simulink model "PID"  (R2020b)
settings: Solver=VariableStepAuto  StartTime=0.0  StopTime=Ts  RelTol=1e-3
values from neighbouring files (symbols this model uses):
  b = 1    [params.m]
  c = 1    [params.m]
  Kc = 3    [params.m]
  Kd = 0.1    [params.m]
  Kff = 1    [params.m]
  Ki = 1    [params.m]
  Kp = 1    [params.m]
  Kpd = 1    [params.m]
  Kpi = 0.2    [params.m]
  Tf = 1    [params.m]
  Tfa1 = 1    [params.m]
  Tfa2 = 1    [params.m]
  Tff1 = 1    [params.m]
  Tff2 = 3    [params.m]
  Ts = 100    [params.m]
  u_max = 5    [params.m]
  u_min = -5    [params.m]
  y_zad = 5    [params.m]
  z_zad = 2    [params.m]
libraries: pid_lib x6
settings Model: Creator=micha  LastModifiedBy=micha
settings DebuggingCC: IgnoredZcDiagnostic=error

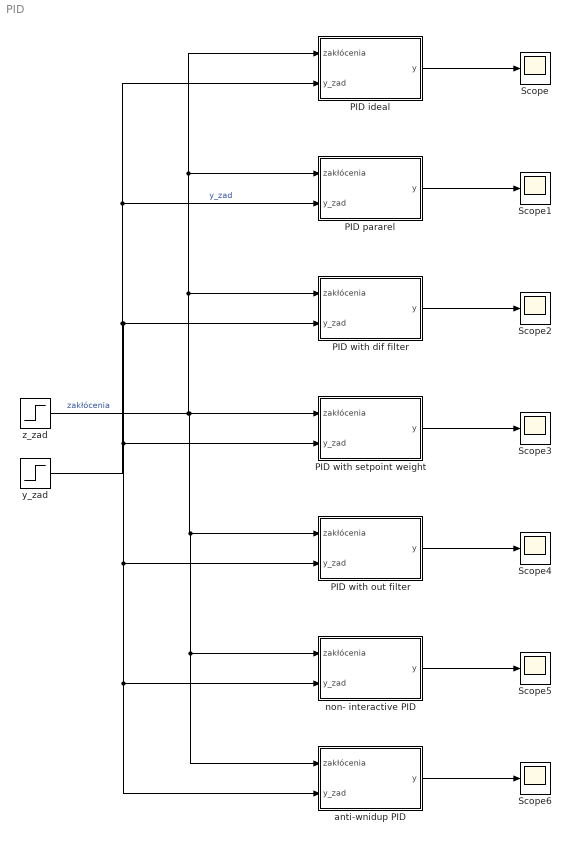
== system PID ==
  PID ideal : Subsystem
  PID pararel : Subsystem
  PID with dif filter : Subsystem
  "PID with out filter " : Subsystem
  PID with setpoint weight : Subsystem
  Scope{,1..6} (7 alike) : Scope
  anti-wnidup PID : Subsystem
  non- interactive PID : Subsystem
  y_zad : Step  After=y_zad  SampleTime=1
  z_zad : Step  Time=50  After=z_zad  SampleTime=1
  wires:
  PID ideal/1(y) -> Scope/1
  PID pararel/1(y) -> Scope1/1
  PID with dif filter/1(y) -> Scope2/1
  PID with setpoint weight/1(y) -> Scope3/1
  "PID with out filter "/1(y) -> Scope4/1
  z_zad/1 -> PID ideal/1(zakłócenia), PID pararel/1(zakłócenia), PID with dif filter/1(zakłócenia), anti-wnidup PID/1(zakłócenia), non- interactive PID/1(zakłócenia), "PID with out filter "/1(zakłócenia), PID with setpoint weight/1(zakłócenia)  "zakłócenia"
  y_zad/1 -> PID ideal/2(y_zad), PID pararel/2(y_zad), anti-wnidup PID/2(y_zad), non- interactive PID/2(y_zad), "PID with out filter "/2(y_zad), PID with setpoint weight/2(y_zad), PID with dif filter/2(y_zad)  "y_zad"
  non- interactive PID/1(y) -> Scope5/1
  anti-wnidup PID/1(y) -> Scope6/1

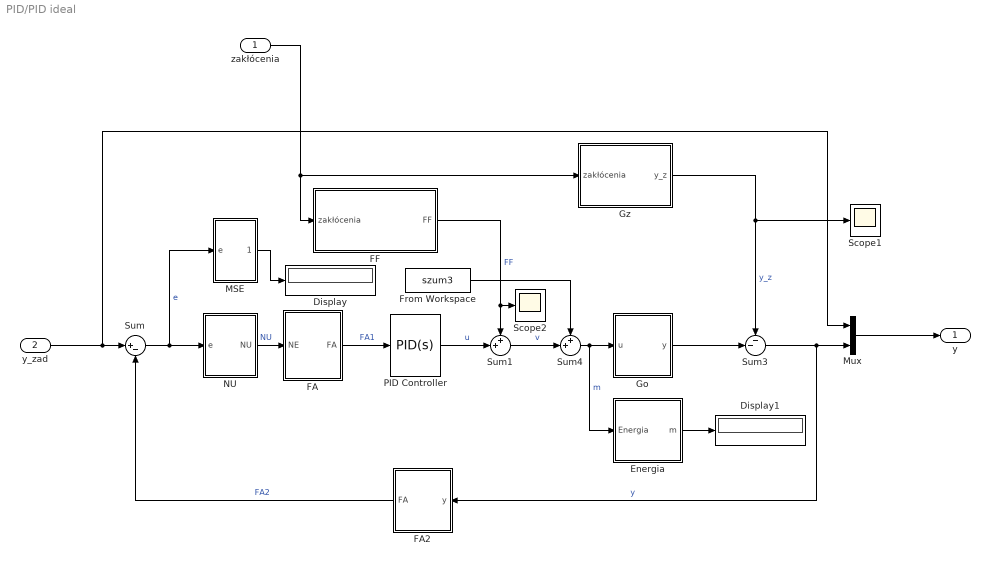
== system PID/PID ideal ==
  zakłócenia : Inport
  y_zad : Inport  Port=2
  Display : Display
  Display1 : Display
  Energia : Subsystem
  FA : Subsystem
  FA2 : Subsystem
  FF : Subsystem
  From Workspace : FromWorkspace  VariableName=szum3  OutDataTypeStr=double  SampleTime=1
  Go : Subsystem
  Gz : Subsystem
  MSE : Subsystem
  Mux : Mux  Inputs=2
  NU : Subsystem
  PID Controller : pid_lib/PID Controller  Controller=PID  Form=Ideal  TimeDomain=Continuous-time  UseExternalTs=off  SampleTime=-1  IntegratorMethod=Forward Euler  FilterMethod=Forward Euler  ControllerParametersSource=internal  P=1.05779168543042  I=0.244759575952049  D=0.993541953243631  UseFilter=on  N=1  TunerSelectOption=Transfer Function Based (PID Tuner App)  InitialConditionSource=internal  InitialConditionForIntegrator=0  InitialConditionForFilter=0  DifferentiatorICPrevScaledInput=0  ExternalReset=none  TrackingMode=off  Kt=1  LimitOutput=off  SatLimitsSource=internal  UpperSaturationLimit=inf  LowerSaturationLimit=-inf  LinearizeAsGain=on  AntiWindupMode=none  Kb=1  POutMin=[]  POutMax=[]  IOutMin=[]  IOutMax=[]  DOutMin=[]  DOutMax=[]  NOutMin=[]  NOutMax=[]  SumOutMin=[]  SumOutMax=[]  SaturationOutMin=[]  SaturationOutMax=[]  PParamMin=[]  PParamMax=[]  IParamMin=[]  IParamMax=[]  DParamMin=[]  DParamMax=[]  NParamMin=[]  NParamMax=[]  KbParamMin=[]  KbParamMax=[]  KtParamMin=[]  KtParamMax=[]  KbOutMin=[]  KbOutMax=[]  KtOutMin=[]  KtOutMax=[]  IntegratorOutMin=[]  IntegratorOutMax=[]  FilterOutMin=[]  FilterOutMax=[]  SumI1OutMin=[]  SumI1OutMax=[]  SumI2OutMin=[]  SumI2OutMax=[]  SumI3OutMin=[]  SumI3OutMax=[]  SumI4OutMin=[]  SumI4OutMax=[]  SumDOutMin=[]  SumDOutMax=[]  DifferentiatorOutMin=[]  DifferentiatorOutMax=[]  FilterDiffOutCoefMin=[]  FilterDiffOutCoefMax=[]  ReciprocalOutMin=[]  ReciprocalOutMax=[]  SumDenOutMin=[]  SumDenOutMax=[]  SumNumOutMin=[]  SumNumOutMax=[]  DivideOutMin=[]  DivideOutMax=[]  UdiffTsProdOutMin=[]  UdiffTsProdOutMax=[]  NTsProdOutMin=[]  NTsProdOutMax=[]  UintegralTsProdOutMin=[]  UintegralTsProdOutMax=[]  UngainTsProdOutMin=[]  UngainTsProdOutMax=[]  IntegratorContinuousStateAttributes=''  IntegratorStateMustResolveToSignalObject=off  IntegratorRTWStateStorageClass=Auto  FilterContinuousStateAttributes=''  FilterStateMustResolveToSignalObject=off  FilterRTWStateStorageClass=Auto  ParallelPVariant=Passthrough  IdealPVariant=InternalParameters  IVariant=InternalParameters  DVariant=InternalParameters  IntegratorVariant=Continuous  SatVariant=Disabled  AWVariant=Passthrough  PCopyVariant=Disabled  TRVariant=Disabled  FdbkBlocksVariant=Forward  IdealPFdbkVariant=Disabled  SatFdbkVariant=Disabled  DerivativeFilterVariant=ContFilter  NVariant=InternalParameters  NCopyVariant=Disabled  FilterICVariant=InternalICsFilter  IntegratorICVariant=InternalICs  ExternalResetVariant=Disabled  TRSumVariant=Passthrough  SumFdbkVariant=Disabled  SumVariant=Sum_PID  TsampFilterVariant=InternalTs  TsampNgainVariant=Passthrough  TsampIntegralVariant=Passthrough  ExternalSaturationOutDataTypeStr=Inherit: Same as second input
  Scope1 : Scope
  Scope2 : Scope
  Sum : Sum  Inputs=|+-
  Sum1 : Sum  Inputs=++|
  Sum3 : Sum  Inputs=--|
  Sum4 : Sum  Inputs=++|
  y : Outport
  wires:
  Sum/1 -> MSE/1(e), NU/1(e)  "e"
  Sum3/1 -> FA2/1(y), Mux/2  "y"
  Gz/1(y_z) -> Scope1/1, Sum3/1  "y_z"
  Energia/1(m) -> Display1/1
  Sum4/1 -> Energia/1(Energia), Go/1(u)  "m"
  zakłócenia/1 -> FF/1(zakłócenia), Gz/1(zakłócenia)
  MSE/1(MSE) -> Display/1
  Go/1(y) -> Sum3/2
  PID Controller/1 -> Sum1/2  "u"
  Sum1/1 -> Sum4/2  "v"
  Mux/1 -> y/1
  y_zad/1 -> Mux/1, Sum/1
  FF/1(FF) -> Scope2/1, Sum1/1  "FF"
  FA/1(FA) -> PID Controller/1  "FA1"
  FA2/1(FA) -> Sum/2  "FA2"
  NU/1(NU) -> FA/1(NE)  "NU"
  From Workspace/1 -> Sum4/1

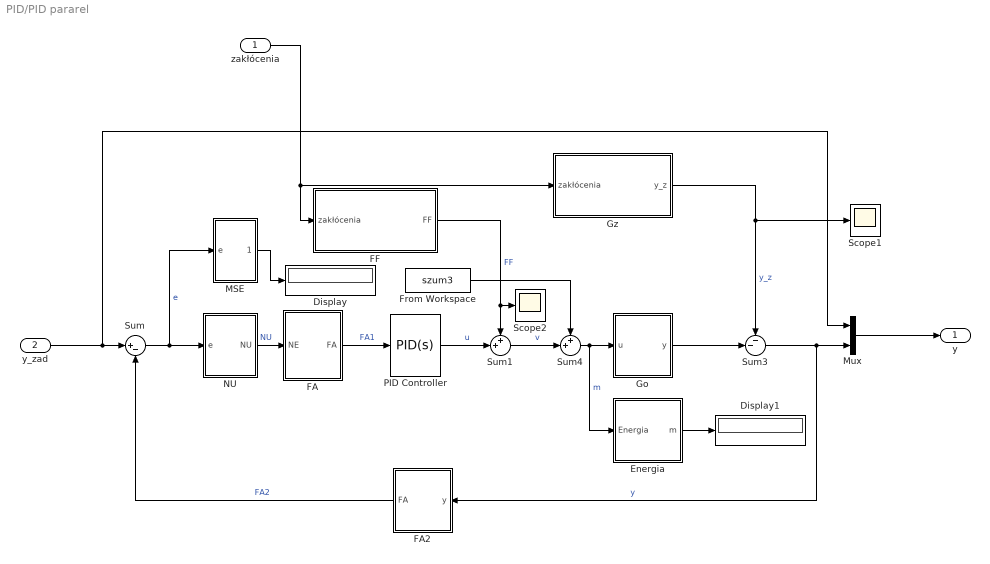
== system PID/PID pararel ==
  zakłócenia : Inport
  y_zad : Inport  Port=2
  Display : Display
  Display1 : Display
  Energia : Subsystem
  FA : Subsystem
  FA2 : Subsystem
  FF : Subsystem
  From Workspace : FromWorkspace  VariableName=szum3  OutDataTypeStr=double  SampleTime=1
  Go : Subsystem
  Gz : Subsystem
  MSE : Subsystem
  Mux : Mux  Inputs=2
  NU : Subsystem
  PID Controller : pid_lib/PID Controller  Controller=PID  Form=Parallel  TimeDomain=Continuous-time  UseExternalTs=off  SampleTime=-1  IntegratorMethod=Forward Euler  FilterMethod=Forward Euler  ControllerParametersSource=internal  P=1.05779168543042  I=0.258904644371552  D=1.05096041726741  UseFilter=on  N=1  TunerSelectOption=Transfer Function Based (PID Tuner App)  InitialConditionSource=internal  InitialConditionForIntegrator=0  InitialConditionForFilter=0  DifferentiatorICPrevScaledInput=0  ExternalReset=none  TrackingMode=off  Kt=1  LimitOutput=off  SatLimitsSource=internal  UpperSaturationLimit=inf  LowerSaturationLimit=-inf  LinearizeAsGain=on  AntiWindupMode=none  Kb=1  POutMin=[]  POutMax=[]  IOutMin=[]  IOutMax=[]  DOutMin=[]  DOutMax=[]  NOutMin=[]  NOutMax=[]  SumOutMin=[]  SumOutMax=[]  SaturationOutMin=[]  SaturationOutMax=[]  PParamMin=[]  PParamMax=[]  IParamMin=[]  IParamMax=[]  DParamMin=[]  DParamMax=[]  NParamMin=[]  NParamMax=[]  KbParamMin=[]  KbParamMax=[]  KtParamMin=[]  KtParamMax=[]  KbOutMin=[]  KbOutMax=[]  KtOutMin=[]  KtOutMax=[]  IntegratorOutMin=[]  IntegratorOutMax=[]  FilterOutMin=[]  FilterOutMax=[]  SumI1OutMin=[]  SumI1OutMax=[]  SumI2OutMin=[]  SumI2OutMax=[]  SumI3OutMin=[]  SumI3OutMax=[]  SumI4OutMin=[]  SumI4OutMax=[]  SumDOutMin=[]  SumDOutMax=[]  DifferentiatorOutMin=[]  DifferentiatorOutMax=[]  FilterDiffOutCoefMin=[]  FilterDiffOutCoefMax=[]  ReciprocalOutMin=[]  ReciprocalOutMax=[]  SumDenOutMin=[]  SumDenOutMax=[]  SumNumOutMin=[]  SumNumOutMax=[]  DivideOutMin=[]  DivideOutMax=[]  UdiffTsProdOutMin=[]  UdiffTsProdOutMax=[]  NTsProdOutMin=[]  NTsProdOutMax=[]  UintegralTsProdOutMin=[]  UintegralTsProdOutMax=[]  UngainTsProdOutMin=[]  UngainTsProdOutMax=[]  IntegratorContinuousStateAttributes=''  IntegratorStateMustResolveToSignalObject=off  IntegratorRTWStateStorageClass=Auto  FilterContinuousStateAttributes=''  FilterStateMustResolveToSignalObject=off  FilterRTWStateStorageClass=Auto  ParallelPVariant=InternalParameters  IdealPVariant=Disabled  IVariant=InternalParameters  DVariant=InternalParameters  IntegratorVariant=Continuous  SatVariant=Disabled  AWVariant=Passthrough  PCopyVariant=Disabled  TRVariant=Disabled  FdbkBlocksVariant=Forward  IdealPFdbkVariant=Disabled  SatFdbkVariant=Disabled  DerivativeFilterVariant=ContFilter  NVariant=InternalParameters  NCopyVariant=Disabled  FilterICVariant=InternalICsFilter  IntegratorICVariant=InternalICs  ExternalResetVariant=Disabled  TRSumVariant=Passthrough  SumFdbkVariant=Disabled  SumVariant=Sum_PID  TsampFilterVariant=InternalTs  TsampNgainVariant=Passthrough  TsampIntegralVariant=Passthrough  ExternalSaturationOutDataTypeStr=Inherit: Same as second input
  Scope1 : Scope
  Scope2 : Scope
  Sum : Sum  Inputs=|+-
  Sum1 : Sum  Inputs=++|
  Sum3 : Sum  Inputs=--|
  Sum4 : Sum  Inputs=++|
  y : Outport
  wires:
  Sum/1 -> MSE/1(e), NU/1(e)  "e"
  Sum3/1 -> FA2/1(y), Mux/2  "y"
  Gz/1(y_z) -> Scope1/1, Sum3/1  "y_z"
  Energia/1(m) -> Display1/1
  From Workspace/1 -> Sum4/1
  Sum4/1 -> Energia/1(Energia), Go/1(u)  "m"
  zakłócenia/1 -> FF/1(zakłócenia), Gz/1(zakłócenia)
  MSE/1(MSE) -> Display/1
  Go/1(y) -> Sum3/2
  PID Controller/1 -> Sum1/2  "u"
  Sum1/1 -> Sum4/2  "v"
  Mux/1 -> y/1
  y_zad/1 -> Mux/1, Sum/1
  FF/1(FF) -> Scope2/1, Sum1/1  "FF"
  FA/1(FA) -> PID Controller/1  "FA1"
  FA2/1(FA) -> Sum/2  "FA2"
  NU/1(NU) -> FA/1(NE)  "NU"

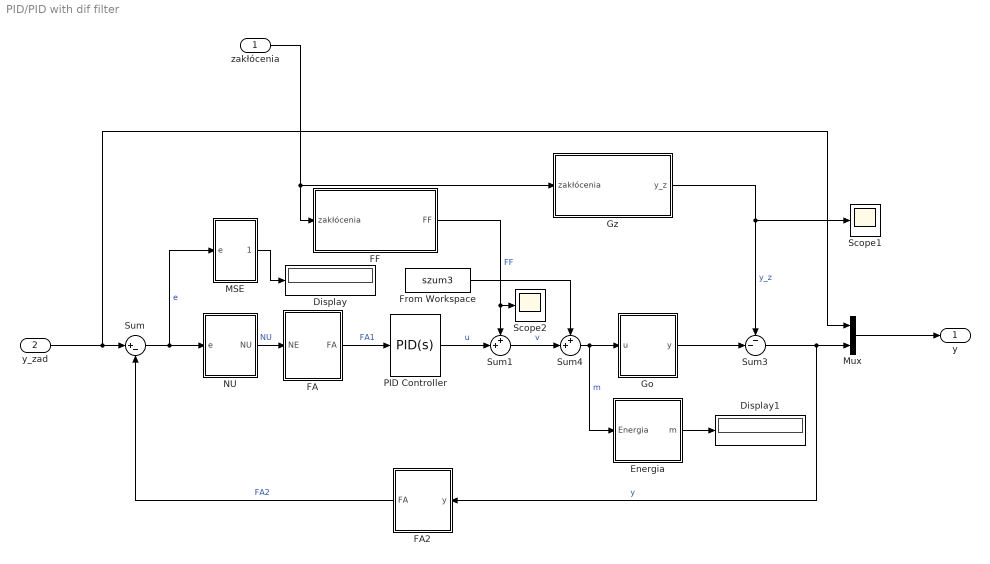
== system PID/PID with dif filter ==
  zakłócenia : Inport
  y_zad : Inport  Port=2
  Display : Display
  Display1 : Display
  Energia : Subsystem
  FA : Subsystem
  FA2 : Subsystem
  FF : Subsystem
  From Workspace : FromWorkspace  VariableName=szum3  OutDataTypeStr=double  SampleTime=1
  Go : Subsystem
  Gz : Subsystem
  MSE : Subsystem
  Mux : Mux  Inputs=2
  NU : Subsystem
  PID Controller : pid_lib/PID Controller  Controller=PID  Form=Ideal  TimeDomain=Continuous-time  UseExternalTs=off  SampleTime=-1  IntegratorMethod=Forward Euler  FilterMethod=Forward Euler  ControllerParametersSource=internal  P=1.05779168543042  I=0.244759575952049  D=0.993541953243631  UseFilter=on  N=49.2140953621087  TunerSelectOption=Transfer Function Based (PID Tuner App)  InitialConditionSource=internal  InitialConditionForIntegrator=0  InitialConditionForFilter=0  DifferentiatorICPrevScaledInput=0  ExternalReset=none  TrackingMode=off  Kt=1  LimitOutput=off  SatLimitsSource=internal  UpperSaturationLimit=inf  LowerSaturationLimit=-inf  LinearizeAsGain=on  AntiWindupMode=none  Kb=1  POutMin=[]  POutMax=[]  IOutMin=[]  IOutMax=[]  DOutMin=[]  DOutMax=[]  NOutMin=[]  NOutMax=[]  SumOutMin=[]  SumOutMax=[]  SaturationOutMin=[]  SaturationOutMax=[]  PParamMin=[]  PParamMax=[]  IParamMin=[]  IParamMax=[]  DParamMin=[]  DParamMax=[]  NParamMin=[]  NParamMax=[]  KbParamMin=[]  KbParamMax=[]  KtParamMin=[]  KtParamMax=[]  KbOutMin=[]  KbOutMax=[]  KtOutMin=[]  KtOutMax=[]  IntegratorOutMin=[]  IntegratorOutMax=[]  FilterOutMin=[]  FilterOutMax=[]  SumI1OutMin=[]  SumI1OutMax=[]  SumI2OutMin=[]  SumI2OutMax=[]  SumI3OutMin=[]  SumI3OutMax=[]  SumI4OutMin=[]  SumI4OutMax=[]  SumDOutMin=[]  SumDOutMax=[]  DifferentiatorOutMin=[]  DifferentiatorOutMax=[]  FilterDiffOutCoefMin=[]  FilterDiffOutCoefMax=[]  ReciprocalOutMin=[]  ReciprocalOutMax=[]  SumDenOutMin=[]  SumDenOutMax=[]  SumNumOutMin=[]  SumNumOutMax=[]  DivideOutMin=[]  DivideOutMax=[]  UdiffTsProdOutMin=[]  UdiffTsProdOutMax=[]  NTsProdOutMin=[]  NTsProdOutMax=[]  UintegralTsProdOutMin=[]  UintegralTsProdOutMax=[]  UngainTsProdOutMin=[]  UngainTsProdOutMax=[]  IntegratorContinuousStateAttributes=''  IntegratorStateMustResolveToSignalObject=off  IntegratorRTWStateStorageClass=Auto  FilterContinuousStateAttributes=''  FilterStateMustResolveToSignalObject=off  FilterRTWStateStorageClass=Auto  ParallelPVariant=Passthrough  IdealPVariant=InternalParameters  IVariant=InternalParameters  DVariant=InternalParameters  IntegratorVariant=Continuous  SatVariant=Disabled  AWVariant=Passthrough  PCopyVariant=Disabled  TRVariant=Disabled  FdbkBlocksVariant=Forward  IdealPFdbkVariant=Disabled  SatFdbkVariant=Disabled  DerivativeFilterVariant=ContFilter  NVariant=InternalParameters  NCopyVariant=Disabled  FilterICVariant=InternalICsFilter  IntegratorICVariant=InternalICs  ExternalResetVariant=Disabled  TRSumVariant=Passthrough  SumFdbkVariant=Disabled  SumVariant=Sum_PID  TsampFilterVariant=InternalTs  TsampNgainVariant=Passthrough  TsampIntegralVariant=Passthrough  ExternalSaturationOutDataTypeStr=Inherit: Same as second input
  Scope1 : Scope
  Scope2 : Scope
  Sum : Sum  Inputs=|+-
  Sum1 : Sum  Inputs=++|
  Sum3 : Sum  Inputs=--|
  Sum4 : Sum  Inputs=++|
  y : Outport
  wires:
  Sum/1 -> MSE/1(e), NU/1(e)  "e"
  Sum3/1 -> FA2/1(y), Mux/2  "y"
  Gz/1(y_z) -> Scope1/1, Sum3/1  "y_z"
  Energia/1(m) -> Display1/1
  From Workspace/1 -> Sum4/1
  Sum4/1 -> Energia/1(Energia), Go/1(u)  "m"
  zakłócenia/1 -> FF/1(zakłócenia), Gz/1(zakłócenia)
  MSE/1(MSE) -> Display/1
  Go/1(y) -> Sum3/2
  PID Controller/1 -> Sum1/2  "u"
  Sum1/1 -> Sum4/2  "v"
  Mux/1 -> y/1
  y_zad/1 -> Mux/1, Sum/1
  FF/1(FF) -> Scope2/1, Sum1/1  "FF"
  FA/1(FA) -> PID Controller/1  "FA1"
  FA2/1(FA) -> Sum/2  "FA2"
  NU/1(NU) -> FA/1(NE)  "NU"

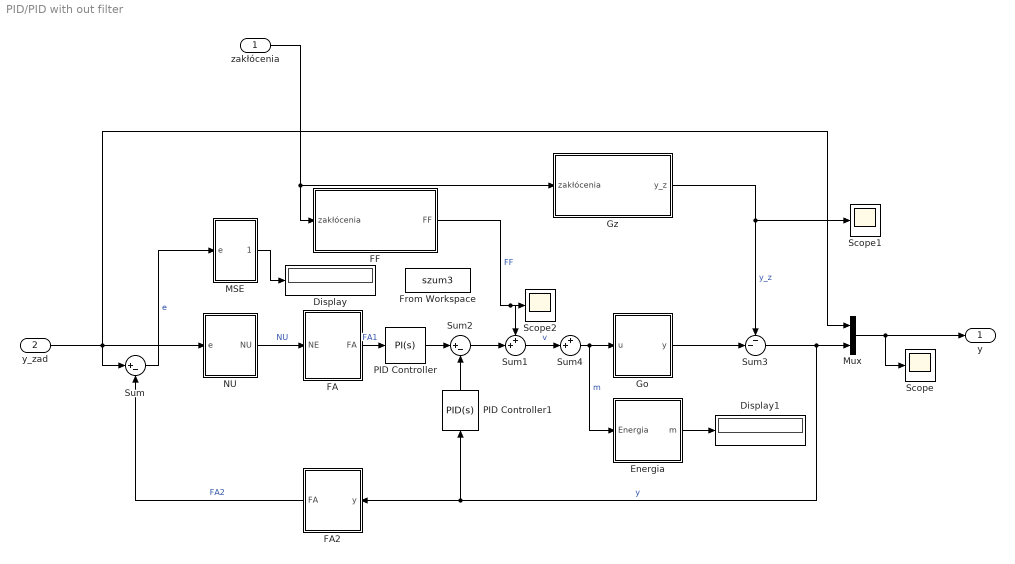
== system PID/PID with out filter  ==
  zakłócenia : Inport
  y_zad : Inport  Port=2
  Display : Display
  Display1 : Display
  Energia : Subsystem
  FA : Subsystem
  FA2 : Subsystem
  FF : Subsystem
  From Workspace : FromWorkspace  VariableName=szum3  OutDataTypeStr=double  SampleTime=1
  Go : Subsystem
  Gz : Subsystem
  MSE : Subsystem
  Mux : Mux  Inputs=2
  NU : Subsystem
  PID Controller : pid_lib/PID Controller  Controller=PI  Form=Parallel  TimeDomain=Continuous-time  UseExternalTs=off  SampleTime=-1  IntegratorMethod=Forward Euler  FilterMethod=Forward Euler  ControllerParametersSource=internal  P=1.5  I=0.38  D=0  UseFilter=on  N=100  TunerSelectOption=Transfer Function Based (PID Tuner App)  InitialConditionSource=internal  InitialConditionForIntegrator=0  InitialConditionForFilter=0  DifferentiatorICPrevScaledInput=0  ExternalReset=none  TrackingMode=off  Kt=1  LimitOutput=off  SatLimitsSource=internal  UpperSaturationLimit=inf  LowerSaturationLimit=-inf  LinearizeAsGain=on  AntiWindupMode=none  Kb=1  POutMin=[]  POutMax=[]  IOutMin=[]  IOutMax=[]  DOutMin=[]  DOutMax=[]  NOutMin=[]  NOutMax=[]  SumOutMin=[]  SumOutMax=[]  SaturationOutMin=[]  SaturationOutMax=[]  PParamMin=[]  PParamMax=[]  IParamMin=[]  IParamMax=[]  DParamMin=[]  DParamMax=[]  NParamMin=[]  NParamMax=[]  KbParamMin=[]  KbParamMax=[]  KtParamMin=[]  KtParamMax=[]  KbOutMin=[]  KbOutMax=[]  KtOutMin=[]  KtOutMax=[]  IntegratorOutMin=[]  IntegratorOutMax=[]  FilterOutMin=[]  FilterOutMax=[]  SumI1OutMin=[]  SumI1OutMax=[]  SumI2OutMin=[]  SumI2OutMax=[]  SumI3OutMin=[]  SumI3OutMax=[]  SumI4OutMin=[]  SumI4OutMax=[]  SumDOutMin=[]  SumDOutMax=[]  DifferentiatorOutMin=[]  DifferentiatorOutMax=[]  FilterDiffOutCoefMin=[]  FilterDiffOutCoefMax=[]  ReciprocalOutMin=[]  ReciprocalOutMax=[]  SumDenOutMin=[]  SumDenOutMax=[]  SumNumOutMin=[]  SumNumOutMax=[]  DivideOutMin=[]  DivideOutMax=[]  UdiffTsProdOutMin=[]  UdiffTsProdOutMax=[]  NTsProdOutMin=[]  NTsProdOutMax=[]  UintegralTsProdOutMin=[]  UintegralTsProdOutMax=[]  UngainTsProdOutMin=[]  UngainTsProdOutMax=[]  IntegratorContinuousStateAttributes=''  IntegratorStateMustResolveToSignalObject=off  IntegratorRTWStateStorageClass=Auto  FilterContinuousStateAttributes=''  FilterStateMustResolveToSignalObject=off  FilterRTWStateStorageClass=Auto  ParallelPVariant=InternalParameters  IdealPVariant=Disabled  IVariant=InternalParameters  DVariant=Disabled  IntegratorVariant=Continuous  SatVariant=Disabled  AWVariant=Passthrough  PCopyVariant=Disabled  TRVariant=Disabled  FdbkBlocksVariant=Forward  IdealPFdbkVariant=Disabled  SatFdbkVariant=Disabled  DerivativeFilterVariant=Disabled  NVariant=Disabled  NCopyVariant=Disabled_SignalSpec  FilterICVariant=Disabled  IntegratorICVariant=InternalICs  ExternalResetVariant=Disabled  TRSumVariant=Passthrough  SumFdbkVariant=Disabled  SumVariant=Sum_PI  TsampFilterVariant=InternalTs  TsampNgainVariant=Passthrough  TsampIntegralVariant=Passthrough  ExternalSaturationOutDataTypeStr=Inherit: Same as second input
  PID Controller1 : pid_lib/PID Controller  Controller=PID  Form=Parallel  TimeDomain=Continuous-time  UseExternalTs=off  SampleTime=-1  IntegratorMethod=Forward Euler  FilterMethod=Forward Euler  ControllerParametersSource=internal  P=0.668790156897551  I=0.381936066634179  D=-0.0850078103169395  UseFilter=on  N=1.08026904337961  TunerSelectOption=Transfer Function Based (PID Tuner App)  InitialConditionSource=internal  InitialConditionForIntegrator=0  InitialConditionForFilter=0  DifferentiatorICPrevScaledInput=0  ExternalReset=none  TrackingMode=off  Kt=1  LimitOutput=off  SatLimitsSource=internal  UpperSaturationLimit=inf  LowerSaturationLimit=-inf  LinearizeAsGain=on  AntiWindupMode=none  Kb=1  POutMin=[]  POutMax=[]  IOutMin=[]  IOutMax=[]  DOutMin=[]  DOutMax=[]  NOutMin=[]  NOutMax=[]  SumOutMin=[]  SumOutMax=[]  SaturationOutMin=[]  SaturationOutMax=[]  PParamMin=[]  PParamMax=[]  IParamMin=[]  IParamMax=[]  DParamMin=[]  DParamMax=[]  NParamMin=[]  NParamMax=[]  KbParamMin=[]  KbParamMax=[]  KtParamMin=[]  KtParamMax=[]  KbOutMin=[]  KbOutMax=[]  KtOutMin=[]  KtOutMax=[]  IntegratorOutMin=[]  IntegratorOutMax=[]  FilterOutMin=[]  FilterOutMax=[]  SumI1OutMin=[]  SumI1OutMax=[]  SumI2OutMin=[]  SumI2OutMax=[]  SumI3OutMin=[]  SumI3OutMax=[]  SumI4OutMin=[]  SumI4OutMax=[]  SumDOutMin=[]  SumDOutMax=[]  DifferentiatorOutMin=[]  DifferentiatorOutMax=[]  FilterDiffOutCoefMin=[]  FilterDiffOutCoefMax=[]  ReciprocalOutMin=[]  ReciprocalOutMax=[]  SumDenOutMin=[]  SumDenOutMax=[]  SumNumOutMin=[]  SumNumOutMax=[]  DivideOutMin=[]  DivideOutMax=[]  UdiffTsProdOutMin=[]  UdiffTsProdOutMax=[]  NTsProdOutMin=[]  NTsProdOutMax=[]  UintegralTsProdOutMin=[]  UintegralTsProdOutMax=[]  UngainTsProdOutMin=[]  UngainTsProdOutMax=[]  IntegratorContinuousStateAttributes=''  IntegratorStateMustResolveToSignalObject=off  IntegratorRTWStateStorageClass=Auto  FilterContinuousStateAttributes=''  FilterStateMustResolveToSignalObject=off  FilterRTWStateStorageClass=Auto  ParallelPVariant=InternalParameters  IdealPVariant=Disabled  IVariant=InternalParameters  DVariant=InternalParameters  IntegratorVariant=Continuous  SatVariant=Disabled  AWVariant=Passthrough  PCopyVariant=Disabled  TRVariant=Disabled  FdbkBlocksVariant=Forward  IdealPFdbkVariant=Disabled  SatFdbkVariant=Disabled  DerivativeFilterVariant=ContFilter  NVariant=InternalParameters  NCopyVariant=Disabled  FilterICVariant=InternalICsFilter  IntegratorICVariant=InternalICs  ExternalResetVariant=Disabled  TRSumVariant=Passthrough  SumFdbkVariant=Disabled  SumVariant=Sum_PID  TsampFilterVariant=InternalTs  TsampNgainVariant=Passthrough  TsampIntegralVariant=Passthrough  ExternalSaturationOutDataTypeStr=Inherit: Same as second input
  Scope : Scope
  Scope1 : Scope
  Scope2 : Scope
  Sum : Sum  Inputs=|+-
  Sum1 : Sum  Inputs=++|
  Sum2 : Sum  Inputs=|+-
  Sum3 : Sum  Inputs=--|
  Sum4 : Sum  Inputs=++|
  y : Outport
  wires:
  Sum/1 -> MSE/1(e)  "e"
  Sum3/1 -> PID Controller1/1, FA2/1(y), Mux/2  "y"
  Gz/1(y_z) -> Scope1/1, Sum3/1  "y_z"
  Energia/1(m) -> Display1/1
  Sum4/1 -> Go/1(u), Energia/1(Energia)  "m"
  zakłócenia/1 -> FF/1(zakłócenia), Gz/1(zakłócenia)
  MSE/1(MSE) -> Display/1
  Go/1(y) -> Sum3/2
  Sum1/1 -> Sum4/2  "v"
  Mux/1 -> Scope/1, y/1
  y_zad/1 -> Mux/1, Sum/1, NU/1(e)
  FF/1(FF) -> Scope2/1, Sum1/1  "FF"
  FA/1(FA) -> PID Controller/1  "FA1"
  FA2/1(FA) -> Sum/2  "FA2"
  NU/1(NU) -> FA/1(NE)  "NU"
  Sum2/1 -> Sum1/2
  PID Controller/1 -> Sum2/1
  PID Controller1/1 -> Sum2/2

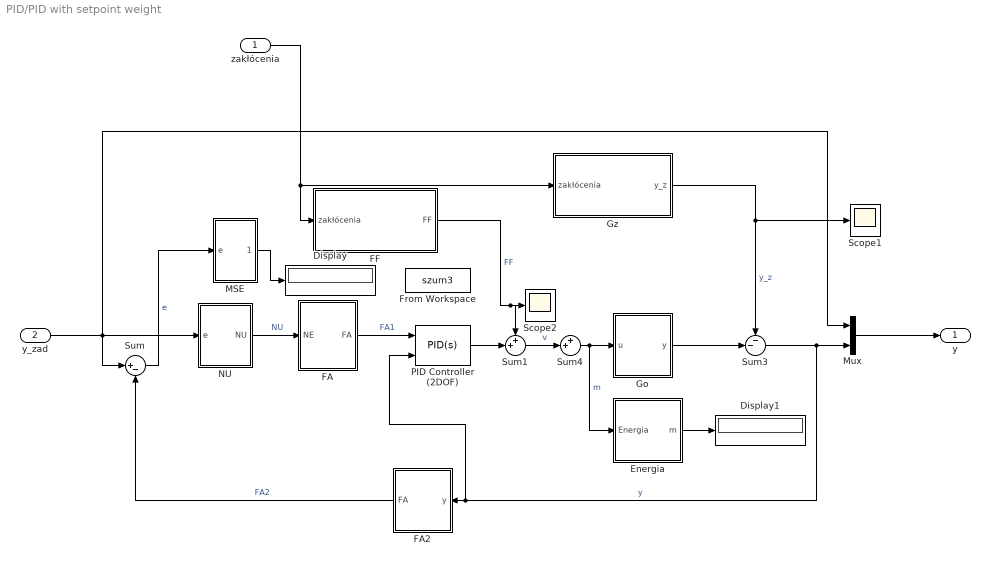
== system PID/PID with setpoint weight ==
  zakłócenia : Inport
  y_zad : Inport  Port=2
  Display : Display
  Display1 : Display
  Energia : Subsystem
  FA : Subsystem
  FA2 : Subsystem
  FF : Subsystem
  From Workspace : FromWorkspace  VariableName=szum3  OutDataTypeStr=double  SampleTime=1
  Go : Subsystem
  Gz : Subsystem
  MSE : Subsystem
  Mux : Mux  Inputs=2
  NU : Subsystem
  PID Controller (2DOF) : pid_lib/PID Controller (2DOF)  Controller=PID  Form=Ideal  TimeDomain=Continuous-time  UseExternalTs=off  SampleTime=-1  IntegratorMethod=Forward Euler  FilterMethod=Forward Euler  ControllerParametersSource=internal  P=0.652114055675395  I=0.613314096005047  D=0  UseFilter=on  N=100  b=1  c=1  TunerSelectOption=Transfer Function Based (PID Tuner App)  InitialConditionSource=internal  InitialConditionForIntegrator=0  InitialConditionForFilter=0  DifferentiatorICPrevScaledInput=0  ExternalReset=none  TrackingMode=off  Kt=1  LimitOutput=off  SatLimitsSource=internal  UpperSaturationLimit=inf  LowerSaturationLimit=-inf  LinearizeAsGain=on  AntiWindupMode=none  Kb=1  POutMin=[]  POutMax=[]  IOutMin=[]  IOutMax=[]  DOutMin=[]  DOutMax=[]  NOutMin=[]  NOutMax=[]  bOutMin=[]  bOutMax=[]  cOutMin=[]  cOutMax=[]  SumOutMin=[]  SumOutMax=[]  SaturationOutMin=[]  SaturationOutMax=[]  PParamMin=[]  PParamMax=[]  IParamMin=[]  IParamMax=[]  DParamMin=[]  DParamMax=[]  NParamMin=[]  NParamMax=[]  bParamMin=[]  bParamMax=[]  cParamMin=[]  cParamMax=[]  KbParamMin=[]  KbParamMax=[]  KtParamMin=[]  KtParamMax=[]  KbOutMin=[]  KbOutMax=[]  KtOutMin=[]  KtOutMax=[]  IntegratorOutMin=[]  IntegratorOutMax=[]  FilterOutMin=[]  FilterOutMax=[]  SumI1OutMin=[]  SumI1OutMax=[]  SumI2OutMin=[]  SumI2OutMax=[]  SumI3OutMin=[]  SumI3OutMax=[]  SumI4OutMin=[]  SumI4OutMax=[]  SumDOutMin=[]  SumDOutMax=[]  Sum1OutMin=[]  Sum1OutMax=[]  Sum2OutMin=[]  Sum2OutMax=[]  Sum3OutMin=[]  Sum3OutMax=[]  DifferentiatorOutMin=[]  DifferentiatorOutMax=[]  FilterDiffOutCoefMin=[]  FilterDiffOutCoefMax=[]  ReciprocalOutMin=[]  ReciprocalOutMax=[]  SumDenOutMin=[]  SumDenOutMax=[]  SumNumOutMin=[]  SumNumOutMax=[]  DivideOutMin=[]  DivideOutMax=[]  UdiffTsProdOutMin=[]  UdiffTsProdOutMax=[]  NTsProdOutMin=[]  NTsProdOutMax=[]  UintegralTsProdOutMin=[]  UintegralTsProdOutMax=[]  UngainTsProdOutMin=[]  UngainTsProdOutMax=[]  IntegratorContinuousStateAttributes=''  IntegratorStateMustResolveToSignalObject=off  IntegratorRTWStateStorageClass=Auto  FilterContinuousStateAttributes=''  FilterStateMustResolveToSignalObject=off  FilterRTWStateStorageClass=Auto  ParallelPVariant=Passthrough  IdealPVariant=InternalParameters  IVariant=InternalParameters  DVariant=InternalParameters  bVariant=InternalParameters  cVariant=InternalParameters  IntegratorVariant=Continuous  SatVariant=Disabled  AWVariant=Passthrough  PCopyVariant=Disabled  TRVariant=Disabled  FdbkBlocksVariant=Forward  IdealPFdbkVariant=Disabled  SatFdbkVariant=Disabled  DerivativeFilterVariant=ContFilter  NVariant=InternalParameters  NCopyVariant=Disabled  FilterICVariant=InternalICsFilter  IntegratorICVariant=InternalICs  ExternalResetVariant=Disabled  TRSumVariant=Passthrough  SumFdbkVariant=Disabled  SumVariant=Sum_PID  TsampFilterVariant=InternalTs  TsampNgainVariant=Passthrough  TsampIntegralVariant=Passthrough  ExternalSaturationOutDataTypeStr=Inherit: Same as second input
      settings: SourceProductBaseCode=SL
  Scope1 : Scope
  Scope2 : Scope
  Sum : Sum  Inputs=|+-
  Sum1 : Sum  Inputs=++|
  Sum3 : Sum  Inputs=--|
  Sum4 : Sum  Inputs=++|
  y : Outport
  wires:
  Sum/1 -> MSE/1(e)  "e"
  Sum3/1 -> PID Controller (2DOF)/2, FA2/1(y), Mux/2  "y"
  Gz/1(y_z) -> Scope1/1, Sum3/1  "y_z"
  Energia/1(m) -> Display1/1
  Sum4/1 -> Energia/1(Energia), Go/1(u)  "m"
  zakłócenia/1 -> FF/1(zakłócenia), Gz/1(zakłócenia)
  MSE/1(MSE) -> Display/1
  Go/1(y) -> Sum3/2
  Sum1/1 -> Sum4/2  "v"
  Mux/1 -> y/1
  y_zad/1 -> Sum/1, NU/1(e), Mux/1
  FF/1(FF) -> Scope2/1, Sum1/1  "FF"
  FA/1(FA) -> PID Controller (2DOF)/1  "FA1"
  FA2/1(FA) -> Sum/2  "FA2"
  NU/1(NU) -> FA/1(NE)  "NU"
  PID Controller (2DOF)/1 -> Sum1/2

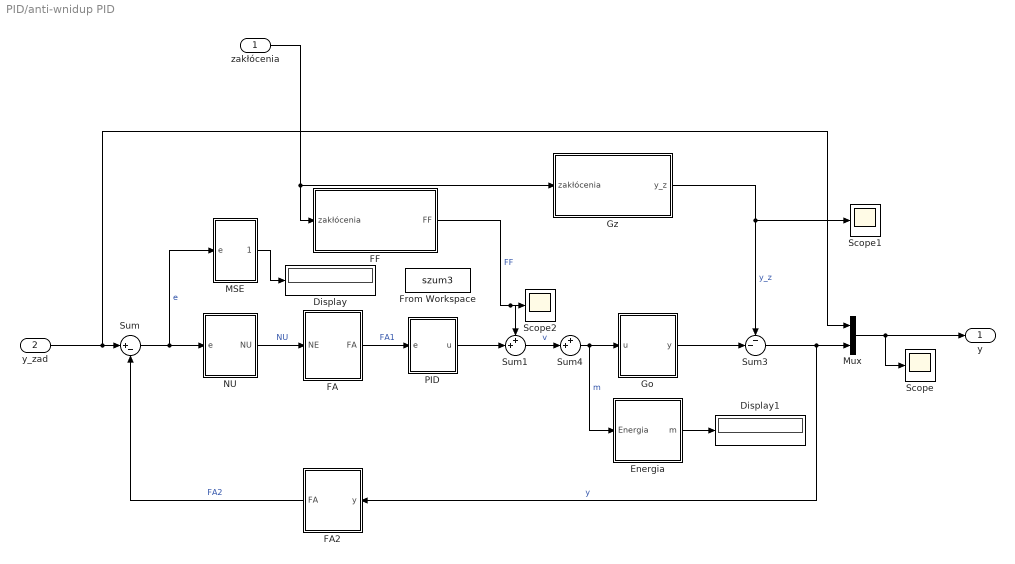
== system PID/anti-wnidup PID ==
  zakłócenia : Inport
  y_zad : Inport  Port=2
  Display : Display
  Display1 : Display
  Energia : Subsystem
  FA : Subsystem
  FA2 : Subsystem
  FF : Subsystem
  From Workspace : FromWorkspace  VariableName=szum3  OutDataTypeStr=double  SampleTime=1
  Go : Subsystem
  Gz : Subsystem
  MSE : Subsystem
  Mux : Mux  Inputs=2
  NU : Subsystem
  PID : Subsystem
  Scope : Scope
  Scope1 : Scope
  Scope2 : Scope
  Sum : Sum  Inputs=|+-
  Sum1 : Sum  Inputs=++|
  Sum3 : Sum  Inputs=--|
  Sum4 : Sum  Inputs=++|
  y : Outport
  wires:
  Sum/1 -> NU/1(e), MSE/1(e)  "e"
  Sum3/1 -> FA2/1(y), Mux/2  "y"
  Gz/1(y_z) -> Scope1/1, Sum3/1  "y_z"
  Energia/1(m) -> Display1/1
  Sum4/1 -> Go/1(u), Energia/1(Energia)  "m"
  zakłócenia/1 -> FF/1(zakłócenia), Gz/1(zakłócenia)
  MSE/1(MSE) -> Display/1
  Sum1/1 -> Sum4/2  "v"
  Mux/1 -> Scope/1, y/1
  y_zad/1 -> Mux/1, Sum/1
  FF/1(FF) -> Scope2/1, Sum1/1  "FF"
  FA/1(FA) -> PID/1(e)  "FA1"
  FA2/1(FA) -> Sum/2  "FA2"
  NU/1(NU) -> FA/1(NE)  "NU"
  PID/1(u) -> Sum1/2
  Go/1(y) -> Sum3/2

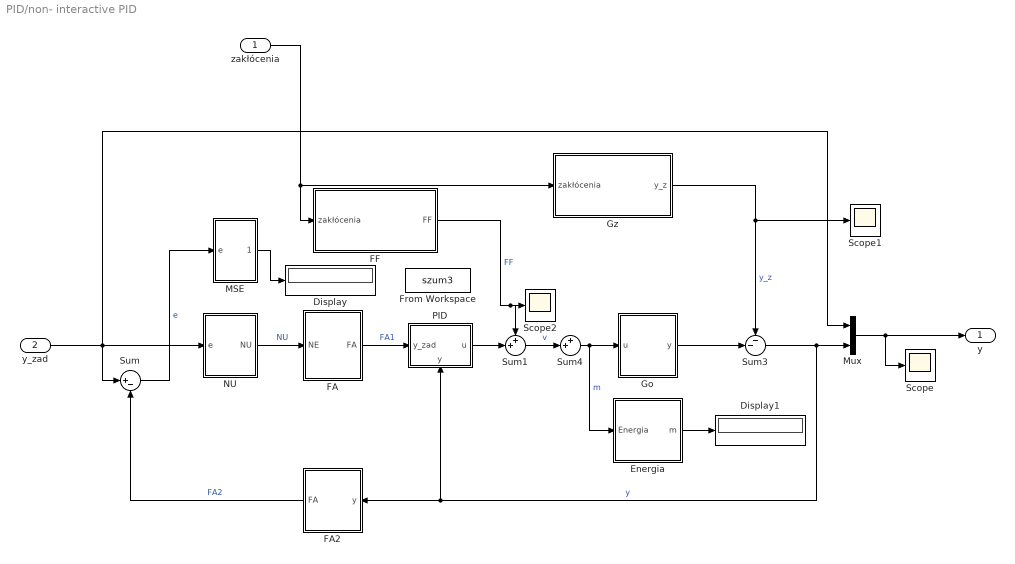
== system PID/non- interactive PID ==
  zakłócenia : Inport
  y_zad : Inport  Port=2
  Display : Display
  Display1 : Display
  Energia : Subsystem
  FA : Subsystem
  FA2 : Subsystem
  FF : Subsystem
  From Workspace : FromWorkspace  VariableName=szum3  OutDataTypeStr=double  SampleTime=1
  Go : Subsystem
  Gz : Subsystem
  MSE : Subsystem
  Mux : Mux  Inputs=2
  NU : Subsystem
  PID : Subsystem
      settings: PortSchema="{\"entries\":[{\"content\":{\"sides\":[{\"content\":{\"connectorIds\":[\"In1\"]},\"type\":\"ConnectorPlacement.EquallySpacedRectSide\",\"uuid\":\"7e1a7a25-6836-4601-abb3-e6db85b28df8\"},{\"content\":{\"connectorIds\":[\"Out1\"],\"side\":\"RIGHT\"},\"type\":\"ConnectorPlacement.EquallySpacedRectSide\",\"uuid\":\"c0dbe357-3eaf-40b5-a51b-245d92cfb79d\"},{\"content\":{\"connectorIds\":[],\"side\":\"TOP\"},\"type\":\"ConnectorPlacement.EquallySpacedRectSide\",\"uuid\":\"e5e97738-3289-4039-b951-83c540cc2e26\"},{\"content\":{\"connectorIds\":[\"In2\"],\"side\":\"BOTTOM\"},\"type\":\"ConnectorPlacement.EquallySpacedRectSide\",\"uuid\":\"b8d19e71-591c-4919-b34a-62c89c6c9aee\"},{\"content\":{\"connectorIds\":[],\"side\":\"HIDDEN\"},\"type\":\"ConnectorPlacement.EquallySpacedRectSide\",\"uuid\":\"5fb2b95d-ebfe-438b-9f91-50160cd846bc\"}]},\"type\":\"ConnectorPlacement.EquallySpacedConnector\",\"uuid\":\"df414232-21c1-425b-aea8-2098730c3b2f\"}],\"packageUris\":[\"http://schema.mathworks.com/mf0/Connector/R2020b\"],\"version\":\"1.0\"}"
  Scope : Scope
  Scope1 : Scope
  Scope2 : Scope
  Sum : Sum  Inputs=|+-
  Sum1 : Sum  Inputs=++|
  Sum3 : Sum  Inputs=--|
  Sum4 : Sum  Inputs=++|
  y : Outport
  wires:
  Sum/1 -> MSE/1(e)  "e"
  Sum3/1 -> PID/2(y), FA2/1(y), Mux/2  "y"
  Gz/1(y_z) -> Scope1/1, Sum3/1  "y_z"
  Energia/1(m) -> Display1/1
  Sum4/1 -> Go/1(u), Energia/1(Energia)  "m"
  zakłócenia/1 -> FF/1(zakłócenia), Gz/1(zakłócenia)
  MSE/1(MSE) -> Display/1
  Go/1(y) -> Sum3/2
  Sum1/1 -> Sum4/2  "v"
  Mux/1 -> Scope/1, y/1
  y_zad/1 -> NU/1(e), Mux/1, Sum/1
  FF/1(FF) -> Scope2/1, Sum1/1  "FF"
  FA/1(FA) -> PID/1(y_zad)  "FA1"
  FA2/1(FA) -> Sum/2  "FA2"
  NU/1(NU) -> FA/1(NE)  "NU"
  PID/1(u) -> Sum1/2

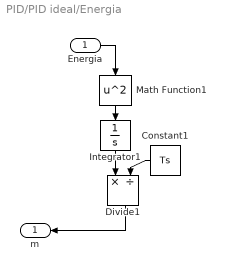
== system PID/PID ideal/Energia ==
  Energia : Inport
  Constant1 : Constant  Value=Ts
  Divide1 : Product  Inputs=*/
  Integrator1 : Integrator
  Math Function1 : Math  Operator=square  SaturateOnIntegerOverflow=on
  m : Outport
  wires:
  Divide1/1 -> m/1
  Integrator1/1 -> Divide1/1
  Math Function1/1 -> Integrator1/1
  Energia/1 -> Math Function1/1
  Constant1/1 -> Divide1/2

== system PID/PID ideal/FA ==
  NE : Inport
  Dead Zone1 : DeadZone  LowerValue=gfa1_lower  UpperValue=gfa1_upper  SaturateOnIntegerOverflow=on
  Transfer Fcn : TransferFcn  Denominator=[Tfa1 1]
  FA : Outport
  wires:
  Dead Zone1/1 -> Transfer Fcn/1
  NE/1 -> Dead Zone1/1
  Transfer Fcn/1 -> FA/1

== system PID/PID ideal/FA2 ==
  y : Inport
  Dead Zone2 : DeadZone  LowerValue=gfa2_lower  UpperValue=gfa2_upper  SaturateOnIntegerOverflow=on
  Transfer Fcn5 : TransferFcn  Denominator=[Tfa2 1]
  FA : Outport
  wires:
  Dead Zone2/1 -> Transfer Fcn5/1
  y/1 -> Dead Zone2/1
  Transfer Fcn5/1 -> FA/1

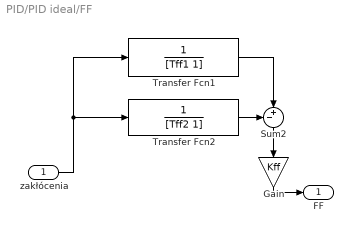
== system PID/PID ideal/FF ==
  zakłócenia : Inport
  Gain : Gain  Gain=Kff
  Sum2 : Sum  Inputs=-+|
  Transfer Fcn1 : TransferFcn  Denominator=[Tff1 1]
  Transfer Fcn2 : TransferFcn  Denominator=[Tff2 1]
  FF : Outport
  wires:
  Transfer Fcn1/1 -> Sum2/2
  zakłócenia/1 -> Transfer Fcn1/1, Transfer Fcn2/1
  Sum2/1 -> Gain/1
  Transfer Fcn2/1 -> Sum2/1
  Gain/1 -> FF/1

== system PID/PID ideal/Go ==
  u : Inport
  Saturation : Saturate  UpperLimit=u_max  LowerLimit=u_min
  Transfer Fcn3 : TransferFcn  Numerator=[-2]  Denominator="[3.5  1]"
  y : Outport
  wires:
  u/1 -> Saturation/1
  Saturation/1 -> Transfer Fcn3/1
  Transfer Fcn3/1 -> y/1

== system PID/PID ideal/Gz ==
  zakłócenia : Inport
  Transfer Fcn4 : TransferFcn  Numerator=[0.8]  Denominator=[21.875 9.75 1]
  Transport Delay : TransportDelay  DelayTime=10
  y_z : Outport
  wires:
  Transport Delay/1 -> y_z/1
  Transfer Fcn4/1 -> Transport Delay/1
  zakłócenia/1 -> Transfer Fcn4/1

== system PID/PID ideal/MSE ==
  e : Inport
  Constant : Constant  Value=Ts
  Divide : Product  Inputs=*/
  Integrator : Integrator
  Math Function : Math  Operator=square  SaturateOnIntegerOverflow=on
  MSE : Outport
  wires:
  Constant/1 -> Divide/2
  e/1 -> Math Function/1
  Math Function/1 -> Integrator/1
  Integrator/1 -> Divide/1
  Divide/1 -> MSE/1

== system PID/PID ideal/NU ==
  e : Inport
  Dead Zone : DeadZone  LowerValue=gnu_lower  UpperValue=gnu_upper  SaturateOnIntegerOverflow=on
  NU : Outport
  wires:
  Dead Zone/1 -> NU/1
  e/1 -> Dead Zone/1

== system PID/PID pararel/Energia ==
  Energia : Inport
  Constant1 : Constant  Value=Ts
  Divide1 : Product  Inputs=*/
  Integrator1 : Integrator
  Math Function1 : Math  Operator=square  SaturateOnIntegerOverflow=on
  m : Outport
  wires:
  Divide1/1 -> m/1
  Integrator1/1 -> Divide1/1
  Math Function1/1 -> Integrator1/1
  Energia/1 -> Math Function1/1
  Constant1/1 -> Divide1/2

== system PID/PID pararel/FA ==
  NE : Inport
  Dead Zone1 : DeadZone  LowerValue=gfa1_lower  UpperValue=gfa1_upper  SaturateOnIntegerOverflow=on
  Transfer Fcn : TransferFcn  Denominator=[Tfa1 1]
  FA : Outport
  wires:
  Dead Zone1/1 -> Transfer Fcn/1
  NE/1 -> Dead Zone1/1
  Transfer Fcn/1 -> FA/1

== system PID/PID pararel/FA2 ==
  y : Inport
  Dead Zone2 : DeadZone  LowerValue=gfa2_lower  UpperValue=gfa2_upper  SaturateOnIntegerOverflow=on
  Transfer Fcn5 : TransferFcn  Denominator=[Tfa2 1]
  FA : Outport
  wires:
  Dead Zone2/1 -> Transfer Fcn5/1
  y/1 -> Dead Zone2/1
  Transfer Fcn5/1 -> FA/1

== system PID/PID pararel/FF ==
  zakłócenia : Inport
  Gain : Gain  Gain=Kff
  Sum2 : Sum  Inputs=-+|
  Transfer Fcn1 : TransferFcn  Denominator=[Tff1 1]
  Transfer Fcn2 : TransferFcn  Denominator=[Tff2 1]
  FF : Outport
  wires:
  Transfer Fcn1/1 -> Sum2/2
  zakłócenia/1 -> Transfer Fcn1/1, Transfer Fcn2/1
  Sum2/1 -> Gain/1
  Transfer Fcn2/1 -> Sum2/1
  Gain/1 -> FF/1

== system PID/PID pararel/Go ==
  u : Inport
  Saturation : Saturate  UpperLimit=u_max  LowerLimit=u_min
  Transfer Fcn3 : TransferFcn  Numerator=[-2]  Denominator="[3.5  1]"
  y : Outport
  wires:
  u/1 -> Saturation/1
  Saturation/1 -> Transfer Fcn3/1
  Transfer Fcn3/1 -> y/1

== system PID/PID pararel/Gz ==
  zakłócenia : Inport
  Transfer Fcn4 : TransferFcn  Numerator=[0.8]  Denominator=[21.875 9.75 1]
  Transport Delay : TransportDelay  DelayTime=10
  y_z : Outport
  wires:
  Transport Delay/1 -> y_z/1
  Transfer Fcn4/1 -> Transport Delay/1
  zakłócenia/1 -> Transfer Fcn4/1

== system PID/PID pararel/MSE ==
  e : Inport
  Constant : Constant  Value=Ts
  Divide : Product  Inputs=*/
  Integrator : Integrator
  Math Function : Math  Operator=square  SaturateOnIntegerOverflow=on
  MSE : Outport
  wires:
  Constant/1 -> Divide/2
  e/1 -> Math Function/1
  Math Function/1 -> Integrator/1
  Integrator/1 -> Divide/1
  Divide/1 -> MSE/1

== system PID/PID pararel/NU ==
  e : Inport
  Dead Zone : DeadZone  LowerValue=gnu_lower  UpperValue=gnu_upper  SaturateOnIntegerOverflow=on
  NU : Outport
  wires:
  Dead Zone/1 -> NU/1
  e/1 -> Dead Zone/1

== system PID/PID with dif filter/Energia ==
  Energia : Inport
  Constant1 : Constant  Value=Ts
  Divide1 : Product  Inputs=*/
  Integrator1 : Integrator
  Math Function1 : Math  Operator=square  SaturateOnIntegerOverflow=on
  m : Outport
  wires:
  Divide1/1 -> m/1
  Integrator1/1 -> Divide1/1
  Math Function1/1 -> Integrator1/1
  Energia/1 -> Math Function1/1
  Constant1/1 -> Divide1/2

== system PID/PID with dif filter/FA ==
  NE : Inport
  Dead Zone1 : DeadZone  LowerValue=gfa1_lower  UpperValue=gfa1_upper  SaturateOnIntegerOverflow=on
  Transfer Fcn : TransferFcn  Denominator=[Tfa1 1]
  FA : Outport
  wires:
  Dead Zone1/1 -> Transfer Fcn/1
  NE/1 -> Dead Zone1/1
  Transfer Fcn/1 -> FA/1

== system PID/PID with dif filter/FA2 ==
  y : Inport
  Dead Zone2 : DeadZone  LowerValue=gfa2_lower  UpperValue=gfa2_upper  SaturateOnIntegerOverflow=on
  Transfer Fcn5 : TransferFcn  Denominator=[Tfa2 1]
  FA : Outport
  wires:
  Dead Zone2/1 -> Transfer Fcn5/1
  y/1 -> Dead Zone2/1
  Transfer Fcn5/1 -> FA/1

== system PID/PID with dif filter/FF ==
  zakłócenia : Inport
  Gain : Gain  Gain=Kff
  Sum2 : Sum  Inputs=-+|
  Transfer Fcn1 : TransferFcn  Denominator=[Tff1 1]
  Transfer Fcn2 : TransferFcn  Denominator=[Tff2 1]
  FF : Outport
  wires:
  Transfer Fcn1/1 -> Sum2/2
  zakłócenia/1 -> Transfer Fcn1/1, Transfer Fcn2/1
  Sum2/1 -> Gain/1
  Transfer Fcn2/1 -> Sum2/1
  Gain/1 -> FF/1

== system PID/PID with dif filter/Go ==
  u : Inport
  Saturation : Saturate  UpperLimit=u_max  LowerLimit=u_min
  Transfer Fcn3 : TransferFcn  Numerator=[-2]  Denominator="[3.5  1]"
  y : Outport
  wires:
  u/1 -> Saturation/1
  Saturation/1 -> Transfer Fcn3/1
  Transfer Fcn3/1 -> y/1

== system PID/PID with dif filter/Gz ==
  zakłócenia : Inport
  Transfer Fcn4 : TransferFcn  Numerator=[0.8]  Denominator=[21.875 9.75 1]
  Transport Delay : TransportDelay  DelayTime=10
  y_z : Outport
  wires:
  Transport Delay/1 -> y_z/1
  Transfer Fcn4/1 -> Transport Delay/1
  zakłócenia/1 -> Transfer Fcn4/1

== system PID/PID with dif filter/MSE ==
  e : Inport
  Constant : Constant  Value=Ts
  Divide : Product  Inputs=*/
  Integrator : Integrator
  Math Function : Math  Operator=square  SaturateOnIntegerOverflow=on
  MSE : Outport
  wires:
  Constant/1 -> Divide/2
  e/1 -> Math Function/1
  Math Function/1 -> Integrator/1
  Integrator/1 -> Divide/1
  Divide/1 -> MSE/1

== system PID/PID with dif filter/NU ==
  e : Inport
  Dead Zone : DeadZone  LowerValue=gnu_lower  UpperValue=gnu_upper  SaturateOnIntegerOverflow=on
  NU : Outport
  wires:
  Dead Zone/1 -> NU/1
  e/1 -> Dead Zone/1

== system PID/PID with out filter /Energia ==
  Energia : Inport
  Constant1 : Constant  Value=Ts
  Divide1 : Product  Inputs=*/
  Integrator1 : Integrator
  Math Function1 : Math  Operator=square  SaturateOnIntegerOverflow=on
  m : Outport
  wires:
  Divide1/1 -> m/1
  Integrator1/1 -> Divide1/1
  Math Function1/1 -> Integrator1/1
  Energia/1 -> Math Function1/1
  Constant1/1 -> Divide1/2

== system PID/PID with out filter /FA ==
  NE : Inport
  Dead Zone1 : DeadZone  LowerValue=gfa1_lower  UpperValue=gfa1_upper  SaturateOnIntegerOverflow=on
  Transfer Fcn : TransferFcn  Denominator=[Tfa1 1]
  FA : Outport
  wires:
  Dead Zone1/1 -> Transfer Fcn/1
  NE/1 -> Dead Zone1/1
  Transfer Fcn/1 -> FA/1

== system PID/PID with out filter /FA2 ==
  y : Inport
  Dead Zone2 : DeadZone  LowerValue=gfa2_lower  UpperValue=gfa2_upper  SaturateOnIntegerOverflow=on
  Transfer Fcn5 : TransferFcn  Denominator=[Tfa2 1]
  FA : Outport
  wires:
  Dead Zone2/1 -> Transfer Fcn5/1
  y/1 -> Dead Zone2/1
  Transfer Fcn5/1 -> FA/1

== system PID/PID with out filter /FF ==
  zakłócenia : Inport
  Gain : Gain  Gain=Kff
  Sum2 : Sum  Inputs=-+|
  Transfer Fcn1 : TransferFcn  Denominator=[Tff1 1]
  Transfer Fcn2 : TransferFcn  Denominator=[Tff2 1]
  FF : Outport
  wires:
  Transfer Fcn1/1 -> Sum2/2
  zakłócenia/1 -> Transfer Fcn1/1, Transfer Fcn2/1
  Sum2/1 -> Gain/1
  Transfer Fcn2/1 -> Sum2/1
  Gain/1 -> FF/1

== system PID/PID with out filter /Go ==
  u : Inport
  Saturation : Saturate  UpperLimit=u_max  LowerLimit=u_min
  Transfer Fcn3 : TransferFcn  Numerator=[-2]  Denominator="[3.5  1]"
  y : Outport
  wires:
  u/1 -> Saturation/1
  Saturation/1 -> Transfer Fcn3/1
  Transfer Fcn3/1 -> y/1

== system PID/PID with out filter /Gz ==
  zakłócenia : Inport
  Transfer Fcn4 : TransferFcn  Numerator=[0.8]  Denominator=[21.875 9.75 1]
  Transport Delay : TransportDelay  DelayTime=10
  y_z : Outport
  wires:
  Transport Delay/1 -> y_z/1
  Transfer Fcn4/1 -> Transport Delay/1
  zakłócenia/1 -> Transfer Fcn4/1

== system PID/PID with out filter /MSE ==
  e : Inport
  Constant : Constant  Value=Ts
  Divide : Product  Inputs=*/
  Integrator : Integrator
  Math Function : Math  Operator=square  SaturateOnIntegerOverflow=on
  MSE : Outport
  wires:
  Constant/1 -> Divide/2
  e/1 -> Math Function/1
  Math Function/1 -> Integrator/1
  Integrator/1 -> Divide/1
  Divide/1 -> MSE/1

== system PID/PID with out filter /NU ==
  e : Inport
  Dead Zone : DeadZone  LowerValue=gnu_lower  UpperValue=gnu_upper  SaturateOnIntegerOverflow=on
  NU : Outport
  wires:
  Dead Zone/1 -> NU/1
  e/1 -> Dead Zone/1

== system PID/PID with setpoint weight/Energia ==
  Energia : Inport
  Constant1 : Constant  Value=Ts
  Divide1 : Product  Inputs=*/
  Integrator1 : Integrator
  Math Function1 : Math  Operator=square  SaturateOnIntegerOverflow=on
  m : Outport
  wires:
  Divide1/1 -> m/1
  Integrator1/1 -> Divide1/1
  Math Function1/1 -> Integrator1/1
  Energia/1 -> Math Function1/1
  Constant1/1 -> Divide1/2

== system PID/PID with setpoint weight/FA ==
  NE : Inport
  Dead Zone1 : DeadZone  LowerValue=gfa1_lower  UpperValue=gfa1_upper  SaturateOnIntegerOverflow=on
  Transfer Fcn : TransferFcn  Denominator=[Tfa1 1]
  FA : Outport
  wires:
  Dead Zone1/1 -> Transfer Fcn/1
  NE/1 -> Dead Zone1/1
  Transfer Fcn/1 -> FA/1

== system PID/PID with setpoint weight/FA2 ==
  y : Inport
  Dead Zone2 : DeadZone  LowerValue=gfa2_lower  UpperValue=gfa2_upper  SaturateOnIntegerOverflow=on
  Transfer Fcn5 : TransferFcn  Denominator=[Tfa2 1]
  FA : Outport
  wires:
  Dead Zone2/1 -> Transfer Fcn5/1
  y/1 -> Dead Zone2/1
  Transfer Fcn5/1 -> FA/1

== system PID/PID with setpoint weight/FF ==
  zakłócenia : Inport
  Gain : Gain  Gain=Kff
  Sum2 : Sum  Inputs=-+|
  Transfer Fcn1 : TransferFcn  Denominator=[Tff1 1]
  Transfer Fcn2 : TransferFcn  Denominator=[Tff2 1]
  FF : Outport
  wires:
  Transfer Fcn1/1 -> Sum2/2
  zakłócenia/1 -> Transfer Fcn1/1, Transfer Fcn2/1
  Sum2/1 -> Gain/1
  Transfer Fcn2/1 -> Sum2/1
  Gain/1 -> FF/1

== system PID/PID with setpoint weight/Go ==
  u : Inport
  Saturation : Saturate  UpperLimit=u_max  LowerLimit=u_min
  Transfer Fcn3 : TransferFcn  Numerator=[-2]  Denominator="[3.5  1]"
  y : Outport
  wires:
  u/1 -> Saturation/1
  Saturation/1 -> Transfer Fcn3/1
  Transfer Fcn3/1 -> y/1

== system PID/PID with setpoint weight/Gz ==
  zakłócenia : Inport
  Transfer Fcn4 : TransferFcn  Numerator=[0.8]  Denominator=[21.875 9.75 1]
  Transport Delay : TransportDelay  DelayTime=10
  y_z : Outport
  wires:
  Transport Delay/1 -> y_z/1
  Transfer Fcn4/1 -> Transport Delay/1
  zakłócenia/1 -> Transfer Fcn4/1

== system PID/PID with setpoint weight/MSE ==
  e : Inport
  Constant : Constant  Value=Ts
  Divide : Product  Inputs=*/
  Integrator : Integrator
  Math Function : Math  Operator=square  SaturateOnIntegerOverflow=on
  MSE : Outport
  wires:
  Constant/1 -> Divide/2
  e/1 -> Math Function/1
  Math Function/1 -> Integrator/1
  Integrator/1 -> Divide/1
  Divide/1 -> MSE/1

== system PID/PID with setpoint weight/NU ==
  e : Inport
  Dead Zone : DeadZone  LowerValue=gnu_lower  UpperValue=gnu_upper  SaturateOnIntegerOverflow=on
  NU : Outport
  wires:
  Dead Zone/1 -> NU/1
  e/1 -> Dead Zone/1

== system PID/anti-wnidup PID/Energia ==
  Energia : Inport
  Constant1 : Constant  Value=Ts
  Divide1 : Product  Inputs=*/
  Integrator1 : Integrator
  Math Function1 : Math  Operator=square  SaturateOnIntegerOverflow=on
  m : Outport
  wires:
  Divide1/1 -> m/1
  Integrator1/1 -> Divide1/1
  Math Function1/1 -> Integrator1/1
  Energia/1 -> Math Function1/1
  Constant1/1 -> Divide1/2

== system PID/anti-wnidup PID/FA ==
  NE : Inport
  Dead Zone1 : DeadZone  LowerValue=gfa1_lower  UpperValue=gfa1_upper  SaturateOnIntegerOverflow=on
  Transfer Fcn : TransferFcn  Denominator=[Tfa1 1]
  FA : Outport
  wires:
  Dead Zone1/1 -> Transfer Fcn/1
  NE/1 -> Dead Zone1/1
  Transfer Fcn/1 -> FA/1

== system PID/anti-wnidup PID/FA2 ==
  y : Inport
  Dead Zone2 : DeadZone  LowerValue=gfa2_lower  UpperValue=gfa2_upper  SaturateOnIntegerOverflow=on
  Transfer Fcn5 : TransferFcn  Denominator=[Tfa2 1]
  FA : Outport
  wires:
  Dead Zone2/1 -> Transfer Fcn5/1
  y/1 -> Dead Zone2/1
  Transfer Fcn5/1 -> FA/1

== system PID/anti-wnidup PID/FF ==
  zakłócenia : Inport
  Gain : Gain  Gain=Kff
  Sum2 : Sum  Inputs=-+|
  Transfer Fcn1 : TransferFcn  Denominator=[Tff1 1]
  Transfer Fcn2 : TransferFcn  Denominator=[Tff2 1]
  FF : Outport
  wires:
  Transfer Fcn1/1 -> Sum2/2
  zakłócenia/1 -> Transfer Fcn1/1, Transfer Fcn2/1
  Sum2/1 -> Gain/1
  Transfer Fcn2/1 -> Sum2/1
  Gain/1 -> FF/1

== system PID/anti-wnidup PID/Go ==
  u : Inport
  Saturation : Saturate  UpperLimit=u_max  LowerLimit=u_min
  Transfer Fcn3 : TransferFcn  Numerator=[-2]  Denominator="[3.5  1]"
  y : Outport
  wires:
  u/1 -> Saturation/1
  Saturation/1 -> Transfer Fcn3/1
  Transfer Fcn3/1 -> y/1

== system PID/anti-wnidup PID/Gz ==
  zakłócenia : Inport
  Transfer Fcn4 : TransferFcn  Numerator=[0.8]  Denominator=[21.875 9.75 1]
  Transport Delay : TransportDelay  DelayTime=10
  y_z : Outport
  wires:
  Transport Delay/1 -> y_z/1
  Transfer Fcn4/1 -> Transport Delay/1
  zakłócenia/1 -> Transfer Fcn4/1

== system PID/anti-wnidup PID/MSE ==
  e : Inport
  Constant : Constant  Value=Ts
  Divide : Product  Inputs=*/
  Integrator : Integrator
  Math Function : Math  Operator=square  SaturateOnIntegerOverflow=on
  MSE : Outport
  wires:
  Constant/1 -> Divide/2
  e/1 -> Math Function/1
  Math Function/1 -> Integrator/1
  Integrator/1 -> Divide/1
  Divide/1 -> MSE/1

== system PID/anti-wnidup PID/NU ==
  e : Inport
  Dead Zone : DeadZone  LowerValue=gnu_lower  UpperValue=gnu_upper  SaturateOnIntegerOverflow=on
  NU : Outport
  wires:
  Dead Zone/1 -> NU/1
  e/1 -> Dead Zone/1

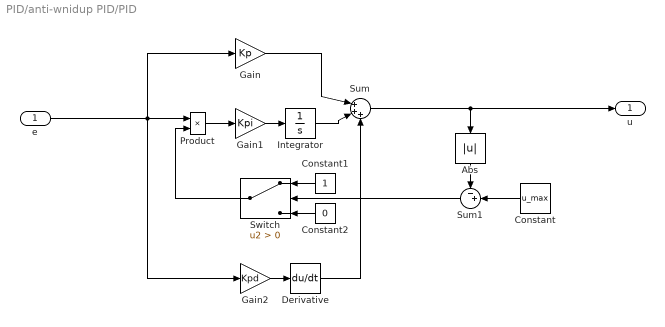
== system PID/anti-wnidup PID/PID ==
  e : Inport
  Abs : Abs
  Constant : Constant  Value=u_max
  Constant1 : Constant
  Constant2 : Constant  Value=0
  Derivative : Derivative
  Gain : Gain  Gain=Kp
  Gain1 : Gain  Gain=Kpi
  Gain2 : Gain  Gain=Kpd
  Integrator : Integrator
  Product : Product
  Sum : Sum  Inputs=|+++
  Sum1 : Sum  Inputs=-+|
  Switch : Switch  Criteria=u2 > Threshold
  u : Outport
  wires:
  Gain/1 -> Sum/1
  e/1 -> Gain/1, Product/1, Gain2/1
  Derivative/1 -> Sum/3
  Integrator/1 -> Sum/2
  Gain2/1 -> Derivative/1
  Gain1/1 -> Integrator/1
  Constant/1 -> Sum1/2
  Sum1/1 -> Switch/2
  Switch/1 -> Product/2
  Constant1/1 -> Switch/1
  Constant2/1 -> Switch/3
  Product/1 -> Gain1/1
  Abs/1 -> Sum1/1
  Sum/1 -> u/1, Abs/1

== system PID/non- interactive PID/Energia ==
  Energia : Inport
  Constant1 : Constant  Value=Ts
  Divide1 : Product  Inputs=*/
  Integrator1 : Integrator
  Math Function1 : Math  Operator=square  SaturateOnIntegerOverflow=on
  m : Outport
  wires:
  Divide1/1 -> m/1
  Integrator1/1 -> Divide1/1
  Math Function1/1 -> Integrator1/1
  Energia/1 -> Math Function1/1
  Constant1/1 -> Divide1/2

== system PID/non- interactive PID/FA ==
  NE : Inport
  Dead Zone1 : DeadZone  LowerValue=gfa1_lower  UpperValue=gfa1_upper  SaturateOnIntegerOverflow=on
  Transfer Fcn : TransferFcn  Denominator=[Tfa1 1]
  FA : Outport
  wires:
  Dead Zone1/1 -> Transfer Fcn/1
  NE/1 -> Dead Zone1/1
  Transfer Fcn/1 -> FA/1

== system PID/non- interactive PID/FA2 ==
  y : Inport
  Dead Zone2 : DeadZone  LowerValue=gfa2_lower  UpperValue=gfa2_upper  SaturateOnIntegerOverflow=on
  Transfer Fcn5 : TransferFcn  Denominator=[Tfa2 1]
  FA : Outport
  wires:
  Dead Zone2/1 -> Transfer Fcn5/1
  y/1 -> Dead Zone2/1
  Transfer Fcn5/1 -> FA/1

== system PID/non- interactive PID/FF ==
  zakłócenia : Inport
  Gain : Gain  Gain=Kff
  Sum2 : Sum  Inputs=-+|
  Transfer Fcn1 : TransferFcn  Denominator=[Tff1 1]
  Transfer Fcn2 : TransferFcn  Denominator=[Tff2 1]
  FF : Outport
  wires:
  Transfer Fcn1/1 -> Sum2/2
  zakłócenia/1 -> Transfer Fcn1/1, Transfer Fcn2/1
  Sum2/1 -> Gain/1
  Transfer Fcn2/1 -> Sum2/1
  Gain/1 -> FF/1

== system PID/non- interactive PID/Go ==
  u : Inport
  Saturation : Saturate  UpperLimit=u_max  LowerLimit=u_min
  Transfer Fcn3 : TransferFcn  Numerator=[-2]  Denominator="[3.5  1]"
  y : Outport
  wires:
  u/1 -> Saturation/1
  Saturation/1 -> Transfer Fcn3/1
  Transfer Fcn3/1 -> y/1

== system PID/non- interactive PID/Gz ==
  zakłócenia : Inport
  Transfer Fcn4 : TransferFcn  Numerator=[0.8]  Denominator=[21.875 9.75 1]
  Transport Delay : TransportDelay  DelayTime=10
  y_z : Outport
  wires:
  Transport Delay/1 -> y_z/1
  Transfer Fcn4/1 -> Transport Delay/1
  zakłócenia/1 -> Transfer Fcn4/1

== system PID/non- interactive PID/MSE ==
  e : Inport
  Constant : Constant  Value=Ts
  Divide : Product  Inputs=*/
  Integrator : Integrator
  Math Function : Math  Operator=square  SaturateOnIntegerOverflow=on
  MSE : Outport
  wires:
  Constant/1 -> Divide/2
  e/1 -> Math Function/1
  Math Function/1 -> Integrator/1
  Integrator/1 -> Divide/1
  Divide/1 -> MSE/1

== system PID/non- interactive PID/NU ==
  e : Inport
  Dead Zone : DeadZone  LowerValue=gnu_lower  UpperValue=gnu_upper  SaturateOnIntegerOverflow=on
  NU : Outport
  wires:
  Dead Zone/1 -> NU/1
  e/1 -> Dead Zone/1

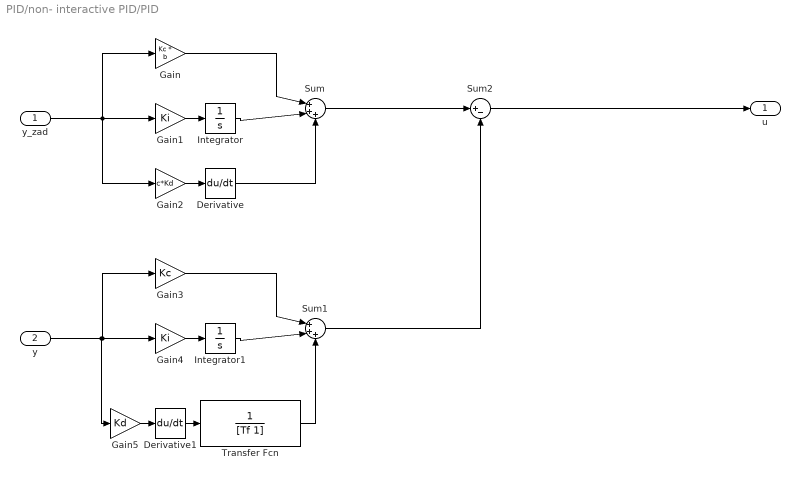
== system PID/non- interactive PID/PID ==
  y_zad : Inport
  y : Inport  Port=2
  Derivative : Derivative
  Derivative1 : Derivative
  Gain : Gain  Gain=Kc * b
  Gain1 : Gain  Gain=Ki
  Gain2 : Gain  Gain=c*Kd
  Gain3 : Gain  Gain=Kc
  Gain4 : Gain  Gain=Ki
  Gain5 : Gain  Gain=Kd
  Integrator : Integrator
  Integrator1 : Integrator
  Sum : Sum  Inputs=|+++
  Sum1 : Sum  Inputs=|+++
  Sum2 : Sum  Inputs=|+-
  Transfer Fcn : TransferFcn  Denominator=[Tf 1]
  u : Outport
  wires:
  y_zad/1 -> Gain/1, Gain2/1, Gain1/1
  Gain1/1 -> Integrator/1
  Gain2/1 -> Derivative/1
  Gain/1 -> Sum/1
  Integrator/1 -> Sum/2
  Derivative/1 -> Sum/3
  Gain3/1 -> Sum1/1
  y/1 -> Gain5/1, Gain3/1, Gain4/1
  Integrator1/1 -> Sum1/2
  Gain4/1 -> Integrator1/1
  Gain5/1 -> Derivative1/1
  Derivative1/1 -> Transfer Fcn/1
  Transfer Fcn/1 -> Sum1/3
  Sum1/1 -> Sum2/2
  Sum/1 -> Sum2/1
  Sum2/1 -> u/1
